simulink model "tilt_quad_sim"  (R2025a)
settings: Solver=ode45  StartTime=0.0  StopTime=sim_time  RelTol=1e-3
values from neighbouring files (symbols this model uses):
  arrive_tol = 0.40    (= 0.4)    [params.m]
  beta_rate_max = deg2rad(45)    [params.m]
  decel_frac = 0.20    (= 0.2)    [params.m]
  descend_rate = 1.2    [params.m]
  Fx_pid_max = 4*Tx_per_rotor    [params.m]
  Fx_pid_min = -Fx_pid_max    [params.m]
  Fz_pid_max = 4*T_max - m*g    (= 45.285)    [params.m]
  Fz_pid_min = -m*g    (= -14.715)    [params.m]
  g = 9.81    [build_model.m]    (also in params.m)
  h_cruise = dg_getvar('h_cruise',  5)    [figure_defs.m]    (also in mission_stats.m = ds_getvar('h_cruise',  5))
  h_land = ds_getvar('h_land',    0)    [mission_stats.m]    (also in params.m = 0)
  h_tol = 0.15    [params.m]
  hover_time = 1.5    [params.m]
  Kd_alt = 8.0    (= 8)    [params.m]
  Kd_phi = 0.4    [params.m]
  Kd_psi = 0.5    [params.m]
  Kd_th = 0.4    [params.m]
  Kd_vx = 0.3    [params.m]
  Ki_alt = 0.8    [params.m]
  Ki_phi = 0.0    (= 0)    [params.m]
  Ki_psi = 0.10    (= 0.1)    [params.m]
  Ki_th = 0.0    (= 0)    [params.m]
  Ki_vx = 0.4    [params.m]
  Kp_alt = 4.0    (= 4)    [params.m]
  Kp_phi = 0.8    [params.m]
  kp_pos_hold = 0.5    [params.m]
  Kp_psi = 1.2    [params.m]
  Kp_th = 0.8    [params.m]
  Kp_vx = 1.5    [params.m]
  m = 1.5    [build_model.m]    (also in params.m)
  min_approach_speed = 0.15    [params.m]
  Mz_pid_max = 6 * k_q * (m*g/4)    (= 0.220725)    [params.m]
  Mz_pid_min = -Mz_pid_max    (= -0.220725)    [params.m]
  Nf_alt = 30    [params.m]
  Nf_att = 30    [params.m]
  Nf_vx = 20    [params.m]
  psi_hold_t = 0.5    [params.m]
  psi_lock_dist = 1.0    (= 1)    [params.m]
  psi_tol = deg2rad(8)    [params.m]
  T_rate_max = 30    [params.m]
  t_takeoff = 8.0    (= 8)    [params.m]
  target_xy = v(:).'; break    [params.m]
  v_cruise = dg_getvar('v_cruise',  8)    [figure_defs.m]    (also in mission_stats.m = ds_getvar('v_cruise',  8))
  v_recover_max = 0.25 * v_cruise    [params.m]
libraries: slpidlib x5
settings Model: Creator=Mias - Laptop  LastModifiedBy=Mias - Laptop

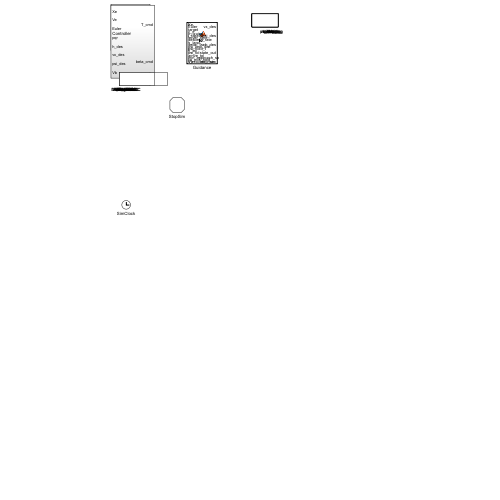
[thumbnail: Simulink's stored preview of the top-level diagram]
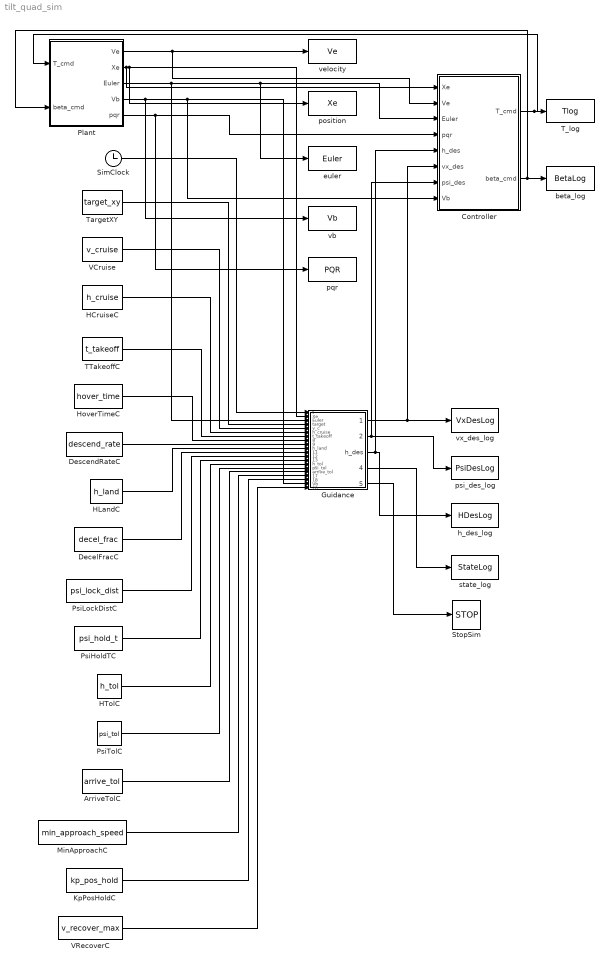
== system tilt_quad_sim ==
  ArriveTolC : Constant  Value=arrive_tol
  Controller : Subsystem
  DecelFracC : Constant  Value=decel_frac
  DescendRateC : Constant  Value=descend_rate
  Guidance : MATLAB Function  TreatAsAtomicUnit=on
  HCruiseC : Constant  Value=h_cruise
  HLandC : Constant  Value=h_land
  HTolC : Constant  Value=h_tol
  HoverTimeC : Constant  Value=hover_time
  KpPosHoldC : Constant  Value=kp_pos_hold
  MinApproachC : Constant  Value=min_approach_speed
  Plant : Subsystem
  PsiHoldTC : Constant  Value=psi_hold_t
  PsiLockDistC : Constant  Value=psi_lock_dist
  PsiTolC : Constant  Value=psi_tol
  SimClock : Clock
  StopSim : Stop
  TTakeoffC : Constant  Value=t_takeoff
  T_log : ToWorkspace  VariableName=Tlog  SaveFormat=Timeseries  SampleTime=-1
  TargetXY : Constant  Value=target_xy
  VCruise : Constant  Value=v_cruise
  VRecoverC : Constant  Value=v_recover_max
  beta_log : ToWorkspace  VariableName=BetaLog  SaveFormat=Timeseries  SampleTime=-1
  euler : ToWorkspace  VariableName=Euler  SaveFormat=Timeseries  SampleTime=-1
  h_des_log : ToWorkspace  VariableName=HDesLog  SaveFormat=Timeseries  SampleTime=-1
  position : ToWorkspace  VariableName=Xe  SaveFormat=Timeseries  SampleTime=-1
  pqr : ToWorkspace  VariableName=PQR  SaveFormat=Timeseries  SampleTime=-1
  psi_des_log : ToWorkspace  VariableName=PsiDesLog  SaveFormat=Timeseries  SampleTime=-1
  state_log : ToWorkspace  VariableName=StateLog  SaveFormat=Timeseries  SampleTime=-1
  vb : ToWorkspace  VariableName=Vb  SaveFormat=Timeseries  SampleTime=-1
  velocity : ToWorkspace  VariableName=Ve  SaveFormat=Timeseries  SampleTime=-1
  vx_des_log : ToWorkspace  VariableName=VxDesLog  SaveFormat=Timeseries  SampleTime=-1
  wires:
  KpPosHoldC/1 -> Guidance/18(kp_pos_hold)
  MinApproachC/1 -> Guidance/17(min_approach_speed)
  Plant/1(Ve) -> Controller/2(Ve), velocity/1
  Plant/2(Xe) -> Guidance/2(Xe), position/1, Controller/1(Xe)
  Plant/3(Euler) -> Controller/3(Euler), euler/1, Guidance/3(Euler)
  Plant/4(Vb) -> Controller/8(Vb), Guidance/19(Vb), vb/1
  HCruiseC/1 -> Guidance/6(h_cruise)
  VCruise/1 -> Guidance/5(v_c)
  Plant/5(pqr) -> Controller/4(pqr), pqr/1
  SimClock/1 -> Guidance/1(t)
  TargetXY/1 -> Guidance/4(target)
  HoverTimeC/1 -> Guidance/8(hover_time)
  TTakeoffC/1 -> Guidance/7(t_takeoff)
  HLandC/1 -> Guidance/10(h_land)
  DescendRateC/1 -> Guidance/9(descend_rate)
  PsiLockDistC/1 -> Guidance/12(psi_lock_dist)
  DecelFracC/1 -> Guidance/11(decel_frac)
  HTolC/1 -> Guidance/14(h_tol)
  PsiHoldTC/1 -> Guidance/13(psi_hold_t)
  ArriveTolC/1 -> Guidance/16(arrive_tol)
  PsiTolC/1 -> Guidance/15(psi_tol)
  VRecoverC/1 -> Guidance/20(v_recover_max)
  Guidance/1(vx_des) -> Controller/6(vx_des), vx_des_log/1
  Guidance/2(psi_des) -> psi_des_log/1, Controller/7(psi_des)
  Guidance/3(h_des) -> Controller/5(h_des), h_des_log/1
  Guidance/4(state_out) -> state_log/1
  Guidance/5(stop_sim) -> StopSim/1
  Controller/1(T_cmd) -> Plant/1(T_cmd), T_log/1
  Controller/2(beta_cmd) -> Plant/2(beta_cmd), beta_log/1

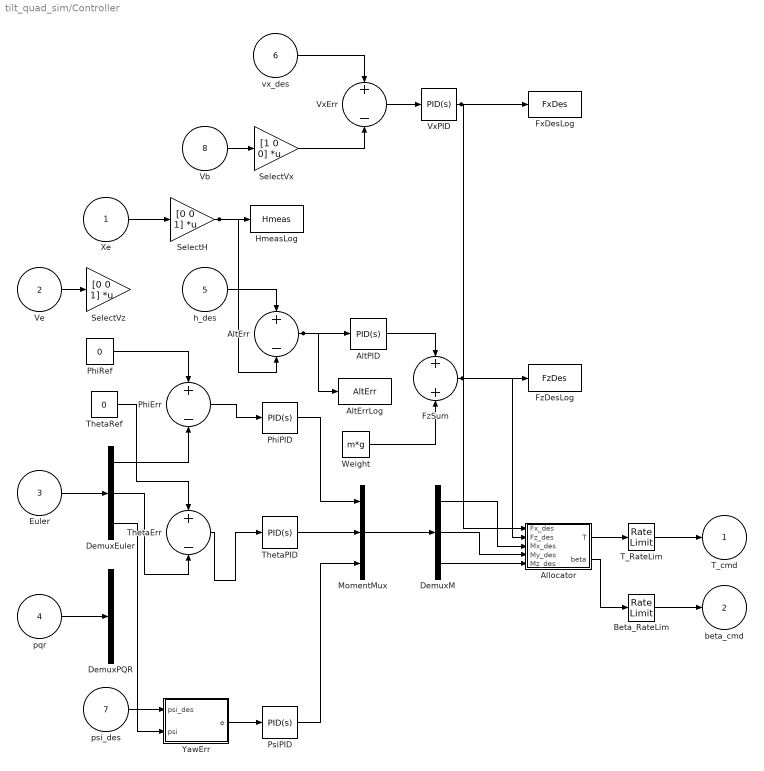
== system tilt_quad_sim/Controller ==
  Xe : Inport
  Ve : Inport  Port=2
  Euler : Inport  Port=3
  pqr : Inport  Port=4
  h_des : Inport  Port=5
  vx_des : Inport  Port=6
  psi_des : Inport  Port=7
  Vb : Inport  Port=8
  Allocator : MATLAB Function  TreatAsAtomicUnit=on
  AltErr : Sum  Inputs=+-
  AltErrLog : ToWorkspace  VariableName=AltErr  SaveFormat=Timeseries  SampleTime=-1
  AltPID : slpidlib/PID Controller  Controller=PID  Form=Parallel  TimeDomain=Continuous-time  UseExternalTs=off  SampleTime=-1  IntegratorMethod=Forward Euler  FilterMethod=Forward Euler  ControllerParametersSource=internal  P=Kp_alt  I=Ki_alt  UseKiTs=off  D=Kd_alt  UseExternalDerivativeSource=off  N=Nf_alt  UseFilter=on  TunerSelectOption=Transfer Function Based (PID Tuner App)  InitialConditionSource=internal  InitialConditionForIntegrator=0  InitialConditionForFilter=0  DifferentiatorICPrevScaledInput=0  ExternalReset=none  TrackingMode=off  Kt=1  LimitOutput=on  SatLimitsSource=internal  UpperSaturationLimit=Fz_pid_max  LowerSaturationLimit=Fz_pid_min  LinearizeAsGain=on  AntiWindupMode=clamping  Kb=1  LimitIntegrator=off  UpperIntegratorSaturationLimit=inf  LowerIntegratorSaturationLimit=-inf  POutMin=[]  POutMax=[]  IOutMin=[]  IOutMax=[]  DOutMin=[]  DOutMax=[]  NOutMin=[]  NOutMax=[]  SumOutMin=[]  SumOutMax=[]  SaturationOutMin=[]  SaturationOutMax=[]  PParamMin=[]  PParamMax=[]  IParamMin=[]  IParamMax=[]  DParamMin=[]  DParamMax=[]  NParamMin=[]  NParamMax=[]  KbParamMin=[]  KbParamMax=[]  KtParamMin=[]  KtParamMax=[]  KbOutMin=[]  KbOutMax=[]  KtOutMin=[]  KtOutMax=[]  IntegratorOutMin=[]  IntegratorOutMax=[]  FilterOutMin=[]  FilterOutMax=[]  SumI1OutMin=[]  SumI1OutMax=[]  SumI2OutMin=[]  SumI2OutMax=[]  SumI3OutMin=[]  SumI3OutMax=[]  SumI4OutMin=[]  SumI4OutMax=[]  SumDOutMin=[]  SumDOutMax=[]  DifferentiatorOutMin=[]  DifferentiatorOutMax=[]  FilterDiffOutCoefMin=[]  FilterDiffOutCoefMax=[]  ReciprocalOutMin=[]  ReciprocalOutMax=[]  SumDenOutMin=[]  SumDenOutMax=[]  SumNumOutMin=[]  SumNumOutMax=[]  DivideOutMin=[]  DivideOutMax=[]  UdiffTsProdOutMin=[]  UdiffTsProdOutMax=[]  NTsProdOutMin=[]  NTsProdOutMax=[]  UintegralTsProdOutMin=[]  UintegralTsProdOutMax=[]  UngainTsProdOutMin=[]  UngainTsProdOutMax=[]  ClampingZeroOutDataTypeStr=Inherit: Inherit via back propagation  ClampingZeroOutMin=[]  ClampingZeroOutMax=[]  FilterDenConstantOutDataTypeStr=Inherit: Inherit via back propagation  FilterDenConstantOutMin=[]  FilterDenConstantOutMax=[]  PCopyOutDataTypeStr=Inherit: Inherit via back propagation  PCopyOutMin=[]  PCopyOutMax=[]  NCopyOutDataTypeStr=Inherit: Inherit via back propagation  NCopyOutMin=[]  NCopyOutMax=[]  IntegratorContinuousStateAttributes=''  IntegratorStateMustResolveToSignalObject=off  IntegratorRTWStateStorageClass=Auto  FilterContinuousStateAttributes=''  FilterStateMustResolveToSignalObject=off  FilterRTWStateStorageClass=Auto  ParallelPVariant=InternalParameters  IdealPVariant=Disabled  IVariant=InternalParameters  DVariant=InternalParameters  IntegratorVariant=Continuous  SatVariant=Enabled  AWVariant=ContClampingParallel  PCopyVariant=Disabled  TRVariant=Disabled  FdbkBlocksVariant=Forward  IdealPFdbkVariant=Disabled  SatFdbkVariant=Disabled  DerivativeFilterVariant=ContFilter  NVariant=InternalParameters  NCopyVariant=Disabled  FilterICVariant=InternalICsFilter  IntegratorICVariant=InternalICs  ExternalResetVariant=Disabled  TRSumVariant=Passthrough  SumFdbkVariant=Disabled  SumVariant=Sum_PID  TsampFilterVariant=InternalTs  TsampNgainVariant=Passthrough  TsampIntegralVariant=Disabled_SignalSpec  ExternalSaturationOutDataTypeStr=Inherit: Same as second input  DerivativeSourceVariant=ErrorSignal  PreIntVariant=InternalPreInt
  Beta_RateLim : RateLimiter  RisingSlewLimit=beta_rate_max  FallingSlewLimit=-beta_rate_max  SampleTimeMode=inherited
  DemuxEuler : Demux  Outputs=3
  DemuxM : Demux  Outputs=3
  DemuxPQR : Demux  Outputs=3
  FxDesLog : ToWorkspace  VariableName=FxDes  SaveFormat=Timeseries  SampleTime=-1
  FzDesLog : ToWorkspace  VariableName=FzDes  SaveFormat=Timeseries  SampleTime=-1
  FzSum : Sum
  HmeasLog : ToWorkspace  VariableName=Hmeas  SaveFormat=Timeseries  SampleTime=-1
  MomentMux : Mux  Inputs=3
  PhiErr : Sum  Inputs=+-
  PhiPID : slpidlib/PID Controller  Controller=PID  Form=Parallel  TimeDomain=Continuous-time  UseExternalTs=off  SampleTime=-1  IntegratorMethod=Forward Euler  FilterMethod=Forward Euler  ControllerParametersSource=internal  P=Kp_phi  I=Ki_phi  UseKiTs=off  D=Kd_phi  UseExternalDerivativeSource=off  N=Nf_att  UseFilter=on  TunerSelectOption=Transfer Function Based (PID Tuner App)  InitialConditionSource=internal  InitialConditionForIntegrator=0  InitialConditionForFilter=0  DifferentiatorICPrevScaledInput=0  ExternalReset=none  TrackingMode=off  Kt=1  LimitOutput=off  SatLimitsSource=internal  UpperSaturationLimit=inf  LowerSaturationLimit=-inf  LinearizeAsGain=on  AntiWindupMode=none  Kb=1  LimitIntegrator=off  UpperIntegratorSaturationLimit=inf  LowerIntegratorSaturationLimit=-inf  POutMin=[]  POutMax=[]  IOutMin=[]  IOutMax=[]  DOutMin=[]  DOutMax=[]  NOutMin=[]  NOutMax=[]  SumOutMin=[]  SumOutMax=[]  SaturationOutMin=[]  SaturationOutMax=[]  PParamMin=[]  PParamMax=[]  IParamMin=[]  IParamMax=[]  DParamMin=[]  DParamMax=[]  NParamMin=[]  NParamMax=[]  KbParamMin=[]  KbParamMax=[]  KtParamMin=[]  KtParamMax=[]  KbOutMin=[]  KbOutMax=[]  KtOutMin=[]  KtOutMax=[]  IntegratorOutMin=[]  IntegratorOutMax=[]  FilterOutMin=[]  FilterOutMax=[]  SumI1OutMin=[]  SumI1OutMax=[]  SumI2OutMin=[]  SumI2OutMax=[]  SumI3OutMin=[]  SumI3OutMax=[]  SumI4OutMin=[]  SumI4OutMax=[]  SumDOutMin=[]  SumDOutMax=[]  DifferentiatorOutMin=[]  DifferentiatorOutMax=[]  FilterDiffOutCoefMin=[]  FilterDiffOutCoefMax=[]  ReciprocalOutMin=[]  ReciprocalOutMax=[]  SumDenOutMin=[]  SumDenOutMax=[]  SumNumOutMin=[]  SumNumOutMax=[]  DivideOutMin=[]  DivideOutMax=[]  UdiffTsProdOutMin=[]  UdiffTsProdOutMax=[]  NTsProdOutMin=[]  NTsProdOutMax=[]  UintegralTsProdOutMin=[]  UintegralTsProdOutMax=[]  UngainTsProdOutMin=[]  UngainTsProdOutMax=[]  ClampingZeroOutDataTypeStr=Inherit: Inherit via back propagation  ClampingZeroOutMin=[]  ClampingZeroOutMax=[]  FilterDenConstantOutDataTypeStr=Inherit: Inherit via back propagation  FilterDenConstantOutMin=[]  FilterDenConstantOutMax=[]  PCopyOutDataTypeStr=Inherit: Inherit via back propagation  PCopyOutMin=[]  PCopyOutMax=[]  NCopyOutDataTypeStr=Inherit: Inherit via back propagation  NCopyOutMin=[]  NCopyOutMax=[]  IntegratorContinuousStateAttributes=''  IntegratorStateMustResolveToSignalObject=off  IntegratorRTWStateStorageClass=Auto  FilterContinuousStateAttributes=''  FilterStateMustResolveToSignalObject=off  FilterRTWStateStorageClass=Auto  ParallelPVariant=InternalParameters  IdealPVariant=Disabled  IVariant=InternalParameters  DVariant=InternalParameters  IntegratorVariant=Continuous  SatVariant=Disabled  AWVariant=Passthrough  PCopyVariant=Disabled  TRVariant=Disabled  FdbkBlocksVariant=Forward  IdealPFdbkVariant=Disabled  SatFdbkVariant=Disabled  DerivativeFilterVariant=ContFilter  NVariant=InternalParameters  NCopyVariant=Disabled  FilterICVariant=InternalICsFilter  IntegratorICVariant=InternalICs  ExternalResetVariant=Disabled  TRSumVariant=Passthrough  SumFdbkVariant=Disabled  SumVariant=Sum_PID  TsampFilterVariant=InternalTs  TsampNgainVariant=Passthrough  TsampIntegralVariant=Disabled_SignalSpec  ExternalSaturationOutDataTypeStr=Inherit: Same as second input  DerivativeSourceVariant=ErrorSignal  PreIntVariant=InternalPreInt
  PhiRef : Constant  Value=0
  PsiPID : slpidlib/PID Controller  Controller=PID  Form=Parallel  TimeDomain=Continuous-time  UseExternalTs=off  SampleTime=-1  IntegratorMethod=Forward Euler  FilterMethod=Forward Euler  ControllerParametersSource=internal  P=Kp_psi  I=Ki_psi  UseKiTs=off  D=Kd_psi  UseExternalDerivativeSource=off  N=Nf_att  UseFilter=on  TunerSelectOption=Transfer Function Based (PID Tuner App)  InitialConditionSource=internal  InitialConditionForIntegrator=0  InitialConditionForFilter=0  DifferentiatorICPrevScaledInput=0  ExternalReset=none  TrackingMode=off  Kt=1  LimitOutput=on  SatLimitsSource=internal  UpperSaturationLimit=Mz_pid_max  LowerSaturationLimit=Mz_pid_min  LinearizeAsGain=on  AntiWindupMode=clamping  Kb=1  LimitIntegrator=off  UpperIntegratorSaturationLimit=inf  LowerIntegratorSaturationLimit=-inf  POutMin=[]  POutMax=[]  IOutMin=[]  IOutMax=[]  DOutMin=[]  DOutMax=[]  NOutMin=[]  NOutMax=[]  SumOutMin=[]  SumOutMax=[]  SaturationOutMin=[]  SaturationOutMax=[]  PParamMin=[]  PParamMax=[]  IParamMin=[]  IParamMax=[]  DParamMin=[]  DParamMax=[]  NParamMin=[]  NParamMax=[]  KbParamMin=[]  KbParamMax=[]  KtParamMin=[]  KtParamMax=[]  KbOutMin=[]  KbOutMax=[]  KtOutMin=[]  KtOutMax=[]  IntegratorOutMin=[]  IntegratorOutMax=[]  FilterOutMin=[]  FilterOutMax=[]  SumI1OutMin=[]  SumI1OutMax=[]  SumI2OutMin=[]  SumI2OutMax=[]  SumI3OutMin=[]  SumI3OutMax=[]  SumI4OutMin=[]  SumI4OutMax=[]  SumDOutMin=[]  SumDOutMax=[]  DifferentiatorOutMin=[]  DifferentiatorOutMax=[]  FilterDiffOutCoefMin=[]  FilterDiffOutCoefMax=[]  ReciprocalOutMin=[]  ReciprocalOutMax=[]  SumDenOutMin=[]  SumDenOutMax=[]  SumNumOutMin=[]  SumNumOutMax=[]  DivideOutMin=[]  DivideOutMax=[]  UdiffTsProdOutMin=[]  UdiffTsProdOutMax=[]  NTsProdOutMin=[]  NTsProdOutMax=[]  UintegralTsProdOutMin=[]  UintegralTsProdOutMax=[]  UngainTsProdOutMin=[]  UngainTsProdOutMax=[]  ClampingZeroOutDataTypeStr=Inherit: Inherit via back propagation  ClampingZeroOutMin=[]  ClampingZeroOutMax=[]  FilterDenConstantOutDataTypeStr=Inherit: Inherit via back propagation  FilterDenConstantOutMin=[]  FilterDenConstantOutMax=[]  PCopyOutDataTypeStr=Inherit: Inherit via back propagation  PCopyOutMin=[]  PCopyOutMax=[]  NCopyOutDataTypeStr=Inherit: Inherit via back propagation  NCopyOutMin=[]  NCopyOutMax=[]  IntegratorContinuousStateAttributes=''  IntegratorStateMustResolveToSignalObject=off  IntegratorRTWStateStorageClass=Auto  FilterContinuousStateAttributes=''  FilterStateMustResolveToSignalObject=off  FilterRTWStateStorageClass=Auto  ParallelPVariant=InternalParameters  IdealPVariant=Disabled  IVariant=InternalParameters  DVariant=InternalParameters  IntegratorVariant=Continuous  SatVariant=Enabled  AWVariant=ContClampingParallel  PCopyVariant=Disabled  TRVariant=Disabled  FdbkBlocksVariant=Forward  IdealPFdbkVariant=Disabled  SatFdbkVariant=Disabled  DerivativeFilterVariant=ContFilter  NVariant=InternalParameters  NCopyVariant=Disabled  FilterICVariant=InternalICsFilter  IntegratorICVariant=InternalICs  ExternalResetVariant=Disabled  TRSumVariant=Passthrough  SumFdbkVariant=Disabled  SumVariant=Sum_PID  TsampFilterVariant=InternalTs  TsampNgainVariant=Passthrough  TsampIntegralVariant=Disabled_SignalSpec  ExternalSaturationOutDataTypeStr=Inherit: Same as second input  DerivativeSourceVariant=ErrorSignal  PreIntVariant=InternalPreInt
  SelectH : Gain  Gain=[0 0 1]  Multiplication=Matrix(K*u)
  SelectVx : Gain  Gain=[1 0 0]  Multiplication=Matrix(K*u)
  SelectVz : Gain  Gain=[0 0 1]  Multiplication=Matrix(K*u)
  T_RateLim : RateLimiter  RisingSlewLimit=T_rate_max  FallingSlewLimit=-T_rate_max  SampleTimeMode=inherited
  ThetaErr : Sum  Inputs=+-
  ThetaPID : slpidlib/PID Controller  Controller=PID  Form=Parallel  TimeDomain=Continuous-time  UseExternalTs=off  SampleTime=-1  IntegratorMethod=Forward Euler  FilterMethod=Forward Euler  ControllerParametersSource=internal  P=Kp_th  I=Ki_th  UseKiTs=off  D=Kd_th  UseExternalDerivativeSource=off  N=Nf_att  UseFilter=on  TunerSelectOption=Transfer Function Based (PID Tuner App)  InitialConditionSource=internal  InitialConditionForIntegrator=0  InitialConditionForFilter=0  DifferentiatorICPrevScaledInput=0  ExternalReset=none  TrackingMode=off  Kt=1  LimitOutput=off  SatLimitsSource=internal  UpperSaturationLimit=inf  LowerSaturationLimit=-inf  LinearizeAsGain=on  AntiWindupMode=none  Kb=1  LimitIntegrator=off  UpperIntegratorSaturationLimit=inf  LowerIntegratorSaturationLimit=-inf  POutMin=[]  POutMax=[]  IOutMin=[]  IOutMax=[]  DOutMin=[]  DOutMax=[]  NOutMin=[]  NOutMax=[]  SumOutMin=[]  SumOutMax=[]  SaturationOutMin=[]  SaturationOutMax=[]  PParamMin=[]  PParamMax=[]  IParamMin=[]  IParamMax=[]  DParamMin=[]  DParamMax=[]  NParamMin=[]  NParamMax=[]  KbParamMin=[]  KbParamMax=[]  KtParamMin=[]  KtParamMax=[]  KbOutMin=[]  KbOutMax=[]  KtOutMin=[]  KtOutMax=[]  IntegratorOutMin=[]  IntegratorOutMax=[]  FilterOutMin=[]  FilterOutMax=[]  SumI1OutMin=[]  SumI1OutMax=[]  SumI2OutMin=[]  SumI2OutMax=[]  SumI3OutMin=[]  SumI3OutMax=[]  SumI4OutMin=[]  SumI4OutMax=[]  SumDOutMin=[]  SumDOutMax=[]  DifferentiatorOutMin=[]  DifferentiatorOutMax=[]  FilterDiffOutCoefMin=[]  FilterDiffOutCoefMax=[]  ReciprocalOutMin=[]  ReciprocalOutMax=[]  SumDenOutMin=[]  SumDenOutMax=[]  SumNumOutMin=[]  SumNumOutMax=[]  DivideOutMin=[]  DivideOutMax=[]  UdiffTsProdOutMin=[]  UdiffTsProdOutMax=[]  NTsProdOutMin=[]  NTsProdOutMax=[]  UintegralTsProdOutMin=[]  UintegralTsProdOutMax=[]  UngainTsProdOutMin=[]  UngainTsProdOutMax=[]  ClampingZeroOutDataTypeStr=Inherit: Inherit via back propagation  ClampingZeroOutMin=[]  ClampingZeroOutMax=[]  FilterDenConstantOutDataTypeStr=Inherit: Inherit via back propagation  FilterDenConstantOutMin=[]  FilterDenConstantOutMax=[]  PCopyOutDataTypeStr=Inherit: Inherit via back propagation  PCopyOutMin=[]  PCopyOutMax=[]  NCopyOutDataTypeStr=Inherit: Inherit via back propagation  NCopyOutMin=[]  NCopyOutMax=[]  IntegratorContinuousStateAttributes=''  IntegratorStateMustResolveToSignalObject=off  IntegratorRTWStateStorageClass=Auto  FilterContinuousStateAttributes=''  FilterStateMustResolveToSignalObject=off  FilterRTWStateStorageClass=Auto  ParallelPVariant=InternalParameters  IdealPVariant=Disabled  IVariant=InternalParameters  DVariant=InternalParameters  IntegratorVariant=Continuous  SatVariant=Disabled  AWVariant=Passthrough  PCopyVariant=Disabled  TRVariant=Disabled  FdbkBlocksVariant=Forward  IdealPFdbkVariant=Disabled  SatFdbkVariant=Disabled  DerivativeFilterVariant=ContFilter  NVariant=InternalParameters  NCopyVariant=Disabled  FilterICVariant=InternalICsFilter  IntegratorICVariant=InternalICs  ExternalResetVariant=Disabled  TRSumVariant=Passthrough  SumFdbkVariant=Disabled  SumVariant=Sum_PID  TsampFilterVariant=InternalTs  TsampNgainVariant=Passthrough  TsampIntegralVariant=Disabled_SignalSpec  ExternalSaturationOutDataTypeStr=Inherit: Same as second input  DerivativeSourceVariant=ErrorSignal  PreIntVariant=InternalPreInt
  ThetaRef : Constant  Value=0
  VxErr : Sum  Inputs=+-
  VxPID : slpidlib/PID Controller  Controller=PID  Form=Parallel  TimeDomain=Continuous-time  UseExternalTs=off  SampleTime=-1  IntegratorMethod=Forward Euler  FilterMethod=Forward Euler  ControllerParametersSource=internal  P=Kp_vx  I=Ki_vx  UseKiTs=off  D=Kd_vx  UseExternalDerivativeSource=off  N=Nf_vx  UseFilter=on  TunerSelectOption=Transfer Function Based (PID Tuner App)  InitialConditionSource=internal  InitialConditionForIntegrator=0  InitialConditionForFilter=0  DifferentiatorICPrevScaledInput=0  ExternalReset=none  TrackingMode=off  Kt=1  LimitOutput=on  SatLimitsSource=internal  UpperSaturationLimit=Fx_pid_max  LowerSaturationLimit=Fx_pid_min  LinearizeAsGain=on  AntiWindupMode=clamping  Kb=1  LimitIntegrator=off  UpperIntegratorSaturationLimit=inf  LowerIntegratorSaturationLimit=-inf  POutMin=[]  POutMax=[]  IOutMin=[]  IOutMax=[]  DOutMin=[]  DOutMax=[]  NOutMin=[]  NOutMax=[]  SumOutMin=[]  SumOutMax=[]  SaturationOutMin=[]  SaturationOutMax=[]  PParamMin=[]  PParamMax=[]  IParamMin=[]  IParamMax=[]  DParamMin=[]  DParamMax=[]  NParamMin=[]  NParamMax=[]  KbParamMin=[]  KbParamMax=[]  KtParamMin=[]  KtParamMax=[]  KbOutMin=[]  KbOutMax=[]  KtOutMin=[]  KtOutMax=[]  IntegratorOutMin=[]  IntegratorOutMax=[]  FilterOutMin=[]  FilterOutMax=[]  SumI1OutMin=[]  SumI1OutMax=[]  SumI2OutMin=[]  SumI2OutMax=[]  SumI3OutMin=[]  SumI3OutMax=[]  SumI4OutMin=[]  SumI4OutMax=[]  SumDOutMin=[]  SumDOutMax=[]  DifferentiatorOutMin=[]  DifferentiatorOutMax=[]  FilterDiffOutCoefMin=[]  FilterDiffOutCoefMax=[]  ReciprocalOutMin=[]  ReciprocalOutMax=[]  SumDenOutMin=[]  SumDenOutMax=[]  SumNumOutMin=[]  SumNumOutMax=[]  DivideOutMin=[]  DivideOutMax=[]  UdiffTsProdOutMin=[]  UdiffTsProdOutMax=[]  NTsProdOutMin=[]  NTsProdOutMax=[]  UintegralTsProdOutMin=[]  UintegralTsProdOutMax=[]  UngainTsProdOutMin=[]  UngainTsProdOutMax=[]  ClampingZeroOutDataTypeStr=Inherit: Inherit via back propagation  ClampingZeroOutMin=[]  ClampingZeroOutMax=[]  FilterDenConstantOutDataTypeStr=Inherit: Inherit via back propagation  FilterDenConstantOutMin=[]  FilterDenConstantOutMax=[]  PCopyOutDataTypeStr=Inherit: Inherit via back propagation  PCopyOutMin=[]  PCopyOutMax=[]  NCopyOutDataTypeStr=Inherit: Inherit via back propagation  NCopyOutMin=[]  NCopyOutMax=[]  IntegratorContinuousStateAttributes=''  IntegratorStateMustResolveToSignalObject=off  IntegratorRTWStateStorageClass=Auto  FilterContinuousStateAttributes=''  FilterStateMustResolveToSignalObject=off  FilterRTWStateStorageClass=Auto  ParallelPVariant=InternalParameters  IdealPVariant=Disabled  IVariant=InternalParameters  DVariant=InternalParameters  IntegratorVariant=Continuous  SatVariant=Enabled  AWVariant=ContClampingParallel  PCopyVariant=Disabled  TRVariant=Disabled  FdbkBlocksVariant=Forward  IdealPFdbkVariant=Disabled  SatFdbkVariant=Disabled  DerivativeFilterVariant=ContFilter  NVariant=InternalParameters  NCopyVariant=Disabled  FilterICVariant=InternalICsFilter  IntegratorICVariant=InternalICs  ExternalResetVariant=Disabled  TRSumVariant=Passthrough  SumFdbkVariant=Disabled  SumVariant=Sum_PID  TsampFilterVariant=InternalTs  TsampNgainVariant=Passthrough  TsampIntegralVariant=Disabled_SignalSpec  ExternalSaturationOutDataTypeStr=Inherit: Same as second input  DerivativeSourceVariant=ErrorSignal  PreIntVariant=InternalPreInt
  Weight : Constant  Value=m*g
  YawErr : MATLAB Function  TreatAsAtomicUnit=on
  T_cmd : Outport
  beta_cmd : Outport  Port=2
  wires:
  ThetaRef/1 -> ThetaErr/1
  Ve/1 -> SelectVz/1
  PsiPID/1 -> MomentMux/3
  Euler/1 -> DemuxEuler/1
  Beta_RateLim/1 -> beta_cmd/1
  T_RateLim/1 -> T_cmd/1
  pqr/1 -> DemuxPQR/1
  Xe/1 -> SelectH/1
  DemuxEuler/3 -> YawErr/2(psi)
  DemuxEuler/2 -> ThetaErr/2
  FzSum/1 -> Allocator/2(Fz_des), FzDesLog/1
  PhiRef/1 -> PhiErr/1
  DemuxEuler/1 -> PhiErr/2
  ThetaErr/1 -> ThetaPID/1
  psi_des/1 -> YawErr/1(psi_des)
  Vb/1 -> SelectVx/1
  SelectH/1 -> AltErr/2, HmeasLog/1
  h_des/1 -> AltErr/1
  PhiErr/1 -> PhiPID/1
  YawErr/1(e) -> PsiPID/1
  vx_des/1 -> VxErr/1
  SelectVx/1 -> VxErr/2
  AltErr/1 -> AltPID/1, AltErrLog/1
  PhiPID/1 -> MomentMux/1
  ThetaPID/1 -> MomentMux/2
  VxErr/1 -> VxPID/1
  AltPID/1 -> FzSum/1
  Weight/1 -> FzSum/2
  MomentMux/1 -> DemuxM/1
  VxPID/1 -> Allocator/1(Fx_des), FxDesLog/1
  DemuxM/3 -> Allocator/5(Mz_des)
  DemuxM/2 -> Allocator/4(My_des)
  DemuxM/1 -> Allocator/3(Mx_des)
  Allocator/1(T) -> T_RateLim/1
  Allocator/2(beta) -> Beta_RateLim/1

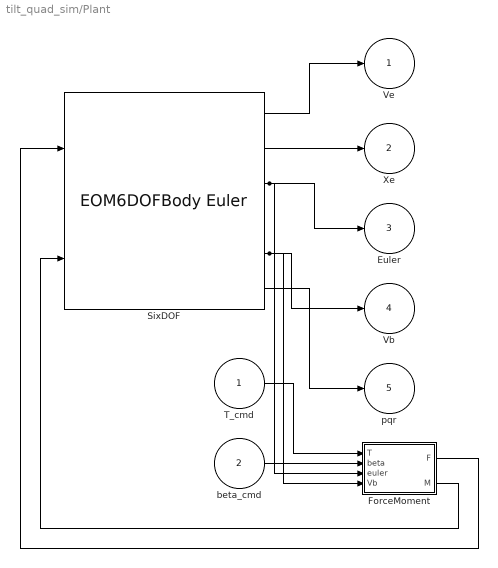
== system tilt_quad_sim/Plant ==
  T_cmd : Inport
  beta_cmd : Inport  Port=2
  ForceMoment : MATLAB Function  TreatAsAtomicUnit=on
  SixDOF : EOM6DOFBodyEuler  mass_0=1.5  inertia=diag([0.02, 0.02, 0.04])
  Ve : Outport
  Xe : Outport  Port=2
  Euler : Outport  Port=3
  Vb : Outport  Port=4
  pqr : Outport  Port=5
  wires:
  SixDOF/1 -> Ve/1
  SixDOF/2 -> Xe/1
  SixDOF/3 -> Euler/1, ForceMoment/3(euler)
  ForceMoment/1(F) -> SixDOF/1
  SixDOF/5 -> Vb/1, ForceMoment/4(Vb)
  SixDOF/6 -> pqr/1
  T_cmd/1 -> ForceMoment/1(T)
  beta_cmd/1 -> ForceMoment/2(beta)
  ForceMoment/2(M) -> SixDOF/2

== matlab function tilt_quad_sim/Controller/YawErr ==
  data: psi_des input; e output; psi input
function e = fcn(psi_des, psi)
%#codegen
d = psi_des - psi;
e = atan2(sin(d), cos(d));
end

== matlab function tilt_quad_sim/Plant/ForceMoment ==
  data: T input; F output; beta input; euler input; Vb input; M output
function [F, M] = fcn(T, beta, euler, Vb)
%#codegen
L = 0.225; k_q = 0.01; m = 1.5; g = 9.81;
r = [ L  L 0; -L  L 0; -L -L 0;  L -L 0];
sgn = [1; -1; 1; -1];
F = zeros(3,1); M = zeros(3,1);
for i = 1:4
  Fi = T(i)*[sin(beta(i)); 0; cos(beta(i))];
  ri = r(i,:).';
  F = F + Fi;
  M = M + cross(ri, Fi);
  M(3) = M(3) + sgn(i)*k_q*T(i)*cos(beta(i));
end
% Rotate gravity from earth frame into body frame using the current Euler angles.
phi = euler(1); theta = euler(2); psi = euler(3);
cph=cos(phi); sph=sin(phi); cth=cos(theta); sth=sin(theta); cps=cos(psi); sps=sin(psi);
R_eb = [ cth*cps,            cth*sps,           -sth;
        sph*sth*cps - cph*sps, sph*sth*sps + cph*cps, sph*cth;
        cph*sth*cps + sph*sps, cph*sth*sps - sph*cps, cph*cth];
g_earth = [0; 0; -g];
g_body  = R_eb * g_earth;
F = F + m * g_body;
% Quadratic drag opposing body velocity — keeps forward flight from accelerating forever.
Cd = [0.05; 0.05; 0.03];
F_drag = -Cd .* Vb .* abs(Vb);
F = F + F_drag;
end

== matlab function tilt_quad_sim/Controller/Allocator ==
  data: Fx_des input; T output; Fz_des input; Mx_des input; My_des input; Mz_des input; beta output
function [T, beta] = fcn(Fx_des, Fz_des, Mx_des, My_des, Mz_des)
%#codegen
L = 0.225; T_max = 15; beta_max = pi/3;
m = 1.5; g = 9.81; eps = 0.0;
k_q = 0.01;  % must match ForceMoment block
% Start with the vertical component each rotor needs to hold altitude
Tz0 = max(Fz_des,0)/4;
% Spread attitude moments via differential vertical thrust
dTz_pitch = My_des / (4*L);
dTz_roll  = Mx_des / (4*L);
% Yaw via reactive-torque differential — pattern [+,-,+,-] matches ForceMoment
dTz_yaw = Mz_des / (4 * k_q);
sgn_pitch     = [-1; +1; +1; -1];
sgn_roll      = [+1; +1; -1; -1];
sgn_yaw_react = [+1; -1; +1; -1];
Tz = Tz0 + sgn_pitch.*dTz_pitch + sgn_roll.*dTz_roll + sgn_yaw_react.*dTz_yaw;
Tz = max(Tz, 0);
% Share forward thrust equally across all four rotors
Tx0 = Fx_des/4;
Tx = Tx0 * ones(4,1);
% Clamp horizontal thrust so no rotor exceeds T_max after combining with vertical
Tx_geom_cap = sqrt(max(T_max^2 - Tz.^2, 0));
for i = 1:4
  if Tx(i) >  Tx_geom_cap(i), Tx(i) =  Tx_geom_cap(i); end
  if Tx(i) < -Tx_geom_cap(i), Tx(i) = -Tx_geom_cap(i); end
end
T  = sqrt(Tx.^2 + Tz.^2);
beta = atan2(Tx, max(Tz,1e-6));
% Hard limits on thrust magnitude and tilt angle
for i = 1:4
  if T(i) > T_max, T(i) = T_max; end
  if T(i) < 0,     T(i) = 0;     end
  if beta(i) >  beta_max, beta(i) =  beta_max; end
  if beta(i) < -beta_max, beta(i) = -beta_max; end
end
end

== matlab function tilt_quad_sim/Guidance ==
  settings: updateMethod=DISCRETE  sampleTime=0.01
  data: t input; vx_des output; Xe input; Euler input; target input; v_c input; h_cruise input; t_takeoff input; hover_time input; descend_rate input; h_land input; decel_frac input; psi_lock_dist input; psi_hold_t input; h_tol input; psi_tol input; arrive_tol input; min_approach_speed input; kp_pos_hold input; Vb input; v_recover_max input; psi_des output; h_des output; state_out output; stop_sim output
function [vx_des, psi_des, h_des, state_out, stop_sim] = fcn(t, Xe, Euler, target, v_c, h_cruise, t_takeoff, hover_time, descend_rate, h_land, decel_frac, psi_lock_dist, psi_hold_t, h_tol, psi_tol, arrive_tol, min_approach_speed, kp_pos_hold, Vb, v_recover_max)
%#codegen
persistent state t_state_entry t_prev psi_locked dist0 h_des_prev t_align_ok t_settle_ok inited
if isempty(inited)
  state = 1; t_state_entry = 0; t_prev = 0;
  psi_locked = Euler(3); dist0 = 1;
  h_des_prev = 0; t_align_ok = -1; t_settle_ok = -1; inited = true;
end
dt = max(t - t_prev, 0);
dx = target(1) - Xe(1);
dy = target(2) - Xe(2);
dist = hypot(dx, dy);
psi_target = atan2(dy, dx);
d = psi_target - Euler(3);
heading_err = atan2(sin(d), cos(d));
h_meas = Xe(3);
vx_des = 0;
psi_des = psi_locked;
h_des = h_des_prev;
switch state
  case 1  % TAKEOFF: ramp altitude using a smoothstep so climb rate is zero at the top
    psi_des = psi_locked;
    if t_takeoff > 0
      tau = min(max((t - t_state_entry) / t_takeoff, 0), 1);
      h_des = h_cruise * (3*tau^2 - 2*tau^3);
    else
      h_des = h_cruise;
    end
    settle_ok = (t - t_state_entry) >= t_takeoff && abs(h_meas - h_cruise) < h_tol && abs(Vb(3)) < 0.15;
    if settle_ok
      if t_settle_ok < 0, t_settle_ok = t; end
    else
      t_settle_ok = -1;
    end
    if t_settle_ok >= 0 && (t - t_settle_ok) >= 1.5
      state = 2; t_state_entry = t; t_align_ok = -1; t_settle_ok = -1;
    end
  case 2  % ALIGN: rotate to face the target before accelerating forward
    psi_des = psi_target;
    h_des = h_cruise;
    if abs(heading_err) < psi_tol
      if t_align_ok < 0, t_align_ok = t; end
    else
      t_align_ok = -1;
    end
    if (t_align_ok >= 0 && (t - t_align_ok) >= psi_hold_t) || (t - t_state_entry) >= 12.0
      state = 3; t_state_entry = t;
      dist0 = max(dist, 1);
      psi_locked = psi_target;
    end
  case 3  % CRUISE: heading frozen; approach with bang-bang braking
    psi_des = psi_locked;
    h_des = h_cruise;
    signed_dist = dx*cos(psi_locked) + dy*sin(psi_locked);
    vbx = Vb(1);
    if signed_dist > 1.5
      a_brake = 3.0;
      stop_d = max(vbx,0)^2 / (2*a_brake);
      if signed_dist > stop_d + 2*arrive_tol
        vx_des = v_c * min((t - t_state_entry)/1.5, 1);  % ease in over 1.5 s to avoid an altitude lurch
      else
        vx_des = 0;
      end
    elseif signed_dist < -1.5
      % Gone past the target — gentle reverse tilt to come back
      vx_des = max(-v_recover_max, kp_pos_hold * signed_dist);
    else
      % Inside the terminal window: P position hold
      vx_des = max(-v_recover_max, min(v_recover_max, kp_pos_hold * signed_dist));
    end
    if (abs(signed_dist) < arrive_tol && abs(vbx) < 0.05) || ((t - t_state_entry) >= 25.0 && abs(signed_dist) < 4*arrive_tol) || ((t - t_state_entry) >= 50.0)
      state = 4; t_state_entry = t;
    end
  case 4  % HOVER: hold position over target for a set dwell time
    psi_des = psi_locked;
    h_des = h_cruise;
    signed_dist = dx*cos(psi_locked) + dy*sin(psi_locked);
    vx_des = max(-0.2, min(0.2, kp_pos_hold * signed_dist));
    if (t - t_state_entry) >= hover_time
      state = 5; t_state_entry = t;
    end
  case 5  % DESCEND: slowly lower altitude while staying above the target
    psi_des = psi_locked;
    h_des = max(h_land, h_des_prev - descend_rate * dt);
    signed_dist = dx*cos(psi_locked) + dy*sin(psi_locked);
    vx_des = max(-0.2, min(0.2, kp_pos_hold * signed_dist));
    if h_des <= h_land + 0.01 || (t - t_state_entry) >= ((h_cruise - h_land)/max(descend_rate,0.05) + 15.0)
      state = 6; t_state_entry = t;
    end
  otherwise  % LANDED: keep the drone softly on the spot
    psi_des = psi_locked;
    h_des = h_land;
    signed_dist = dx*cos(psi_locked) + dy*sin(psi_locked);
    vx_des = max(-0.15, min(0.15, kp_pos_hold * signed_dist));
end
h_des_prev = h_des;
t_prev = t;
state_out = double(state);
stop_sim = double(state == 6 && (t - t_state_entry) >= 6.0);
end
